simulink model "Combined_cycle"  (R2024b)
settings: Solver=VariableStepAuto  StartTime=0.0  StopTime=50  RelTol=1e-3
settings Model: Creator=HP  LastModifiedBy=Ioannis Vourkas

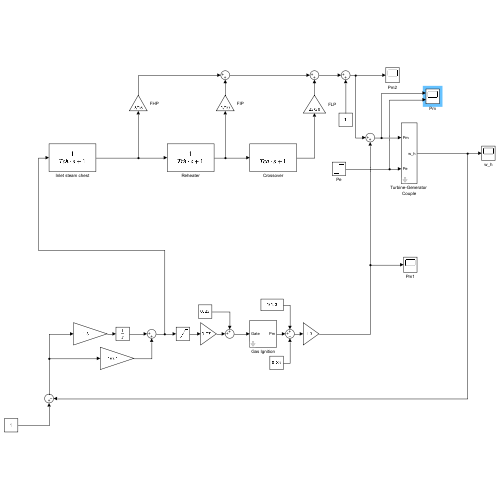
[thumbnail: Simulink's stored preview of the top-level diagram]
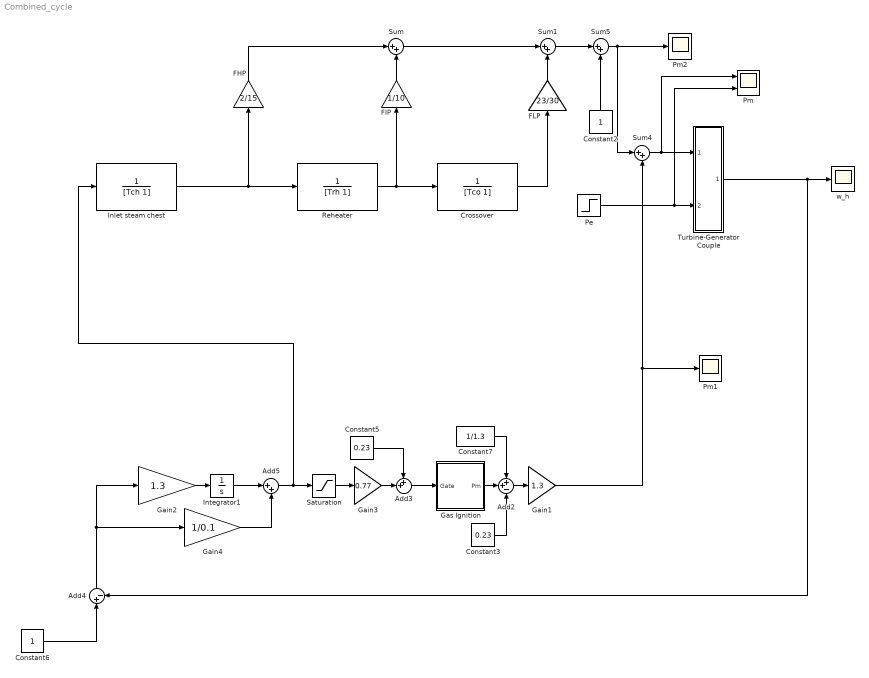
== system Combined_cycle ==
  Add2 : Sum  Inputs=++-
  Add3 : Sum  Inputs=++|
  Add4 : Sum  Inputs=|+-
  Add5 : Sum  Inputs=|++
  Constant2 : Constant
  Constant3 : Constant  Value=0.23
  Constant5 : Constant  Value=0.23
  Constant6 : Constant
  Constant7 : Constant  Value=1/1.3
  Crossover : TransferFcn  Denominator=[Tco 1]  mask{Tco=13/30}
      mask prompts: Tco "Crossover Time Constant / Low-Pressure (LP) Turbine Time Constant)"
      mask DialogControl ParameterGroupVar Prompt: Parameters
  FHP : Gain  Gain=2/15
  FIP : Gain  Gain=1/10
  FLP : Gain  Gain=23/30
  Gain1 : Gain  Gain=1.3
  Gain2 : Gain  Gain=1.3
  Gain3 : Gain  Gain=0.77
  Gain4 : Gain  Gain=1/0.1
  Gas Ignition : Subsystem  mask{Tw=0.4, ini=0.23+1/1.3}
      mask prompts: Tw "Gas ignition constant"; ini "Initial Pm"
  Inlet steam chest : TransferFcn  Denominator=[Tch 1]  mask{Tch=1/10}
      mask prompts: Tch "HP cynlinder time constant"
      mask DialogControl ParameterGroupVar Prompt: Parameters
  Integrator1 : Integrator
  Pe : Step  Time=5  Before=2  After=3  SampleTime=0
  Pm : Scope  NumInputPorts=2
  Pm1 : Scope
  Pm2 : Scope
  Reheater : TransferFcn  Denominator=[Trh 1]  mask{Trh=23/30}
      mask prompts: Trh "Reheater Time Constant"
      mask DialogControl ParameterGroupVar Prompt: Parameters
  Saturation : Saturate  UpperLimit=0.8  LowerLimit=-0.8
  Sum{,1,4..5} (4 alike) : Sum  Inputs=|++
  Turbine-Generator Couple : Subsystem  mask{Hh=20, w_ini=1}
      mask prompts: Hh "H/E Inertia Constant"; w_ini "Initial omega"
  w_h : Scope
  wires:
  Add2/1 -> Gain1/1
  Gas Ignition/1(Pm) -> Add2/2
  Constant6/1 -> Add4/1
  Gain1/1 -> Sum4/2, Pm1/1
  Saturation/1 -> Gain3/1
  Constant7/1 -> Add2/1
  Constant3/1 -> Add2/3
  Constant5/1 -> Add3/1
  Add3/1 -> Gas Ignition/1(Gate)
  Gain3/1 -> Add3/2
  Crossover/1 -> FLP/1
  FLP/1 -> Sum1/2
  Sum/1 -> Sum1/1
  FHP/1 -> Sum/1
  Reheater/1 -> Crossover/1, FIP/1
  Inlet steam chest/1 -> FHP/1, Reheater/1
  Turbine-Generator Couple/1(w_h) -> Add4/2, w_h/1
  FIP/1 -> Sum/2
  Sum4/1 -> Pm/1, Turbine-Generator Couple/1(Pm)
  Pe/1 -> Pm/2, Turbine-Generator Couple/2(Pe)
  Sum1/1 -> Sum5/1
  Constant2/1 -> Sum5/2
  Sum5/1 -> Sum4/1, Pm2/1
  Gain4/1 -> Add5/2
  Integrator1/1 -> Add5/1
  Gain2/1 -> Integrator1/1
  Add5/1 -> Inlet steam chest/1, Saturation/1
  Add4/1 -> Gain2/1, Gain4/1

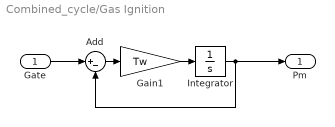
== system Combined_cycle/Gas Ignition ==
  Gate : Inport
  Add : Sum  Inputs=|+-
  Gain1 : Gain  Gain=Tw
  Integrator : Integrator  InitialCondition=0.23
  Pm : Outport
  wires:
  Gain1/1 -> Integrator/1
  Add/1 -> Gain1/1
  Integrator/1 -> Pm/1, Add/2
  Gate/1 -> Add/1

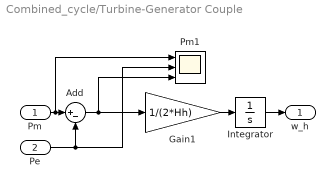
== system Combined_cycle/Turbine-Generator Couple ==
  Pm : Inport
  Pe : Inport  Port=2
  Add : Sum  Inputs=|+-
  Gain1 : Gain  Gain=1/(2*Hh)
  Integrator : Integrator  InitialCondition=w_ini
  Pm1 : Scope  NumInputPorts=3
  w_h : Outport
  wires:
  Pm/1 -> Pm1/1, Add/1
  Gain1/1 -> Integrator/1
  Integrator/1 -> w_h/1
  Add/1 -> Pm1/3, Gain1/1
  Pe/1 -> Add/2, Pm1/2
